simulink library "brk"  (Simulink 8.1)
settings: Solver=ode45  StartTime=0.0  StopTime=10.0  RelTol=1e-3
undefined symbols (not defined in the file or in its folder): KIFO_BrakePressureLimit_bar
settings Model: Creator=xsellart  LastModifiedBy=AT015555

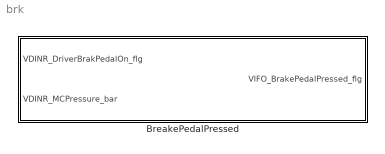
== system brk ==
  BreakePedalPressed : Subsystem

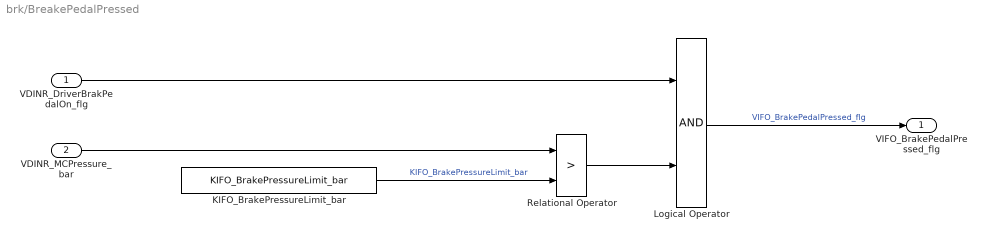
== system brk/BreakePedalPressed ==
  VDINR_DriverBrakPedalOn_flg : Inport
  VDINR_MCPressure_bar : Inport  Port=2
  KIFO_BrakePressureLimit_bar : Constant  Value=KIFO_BrakePressureLimit_bar  OutDataTypeStr=single
  Logical Operator : Logic  AllPortsSameDT=off  OutDataTypeStr=boolean
  Relational Operator : RelationalOperator  Operator=>  OutDataTypeStr=boolean
  VIFO_BrakePedalPressed_flg : Outport
  wires:
  VDINR_MCPressure_bar/1 -> Relational Operator/1
  KIFO_BrakePressureLimit_bar/1 -> Relational Operator/2  "KIFO_BrakePressureLimit_bar"
  VDINR_DriverBrakPedalOn_flg/1 -> Logical Operator/1
  Relational Operator/1 -> Logical Operator/2
  Logical Operator/1 -> VIFO_BrakePedalPressed_flg/1  "VIFO_BrakePedalPressed_flg"
